simulink model "torque_pi_controller_incremental_algorithm_hardware"  (R2023b)
settings: Solver=FixedStepAuto  StartTime=0.0  StopTime=3.5  RelTol=1e-5  EnableMultiTasking=on
values from neighbouring files (symbols this model uses):
  K = 1.339    [torque_PI_integral_algorithm.m]    (also in torque_PI_tuning.m; torque_model.m = 1.32)
  Kp = pid.Kp    [torque_PI_integral_algorithm.m]    (also in torque_PI_tuning.m = G_T*Ki)
  Ti = pid.Ti    [torque_PI_integral_algorithm.m]    (also in torque_PI_tuning.m = Kp/Ki)
  Ts = 0.005    [torque_PI_integral_algorithm.m]    (also in torque_PI_tuning.m)
undefined symbols (not defined in the file or in its folder): DiscIntNeverNeededParam
settings Model: ExtModeTrigDuration=10  Creator=paoli  LastModifiedBy=kiraa
settings OptimizationCC: EnhancedBackFolding=on  PassReuseOutputArgsAs=Individual arguments  ZeroExternalMemoryAtStartup=off  ZeroInternalMemoryAtStartup=off  MaxStackSize=64  OptimizeBlockOrder=speed  DifferentSizesBufferReuse=on  OptimizationCustomize=off  EfficientTunableParamExpr=on
settings DebuggingCC: ParameterTunabilityLossMsg=error
settings HardwareCC: ProdBitPerPointer=32  ProdBitPerSizeT=32  ProdBitPerPtrDiffT=32  ProdLargestAtomicInteger=Long  ProdLargestAtomicFloat=Double  ProdWordSize=32  ProdLongLongMode=on  ProdHWDeviceType=ARM Compatible->ARM Cortex
settings SFSimCC: MATLABDynamicMemAlloc=off
settings RTWCC: Description=Embedded Coder  SystemTargetFile=ert.tlc  HardwareBoard=STM32 Nucleo F401RE  TemplateMakefile=ert_default_tmf  Toolchain=GNU Tools for ARM Embedded Processors
settings CodeAppCC: ForceParamTrailComments=on  IgnoreCustomStorageClasses=off  OperatorAnnotations=on  SimulinkDataObjDesc=on  SFDataObjDesc=on  InsertBlockDesc=on
settings ERTTargetCC: ExtModeTransport=3  ExtModeStaticAlloc=on  ExtModeStaticAllocSize=2000  ExtModeMexFile=ext_xcp  ExtModeIntrfLevel=Level2 - Open

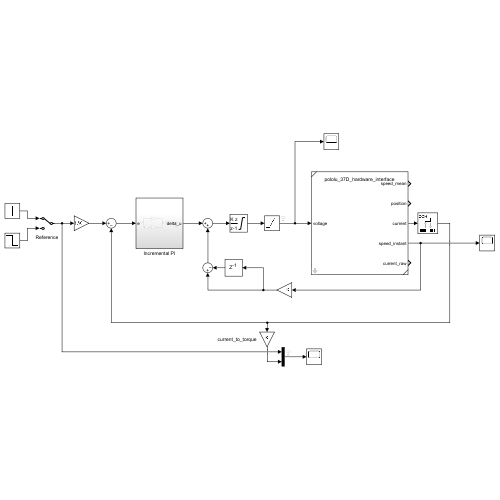
[thumbnail: Simulink's stored preview of the top-level diagram]
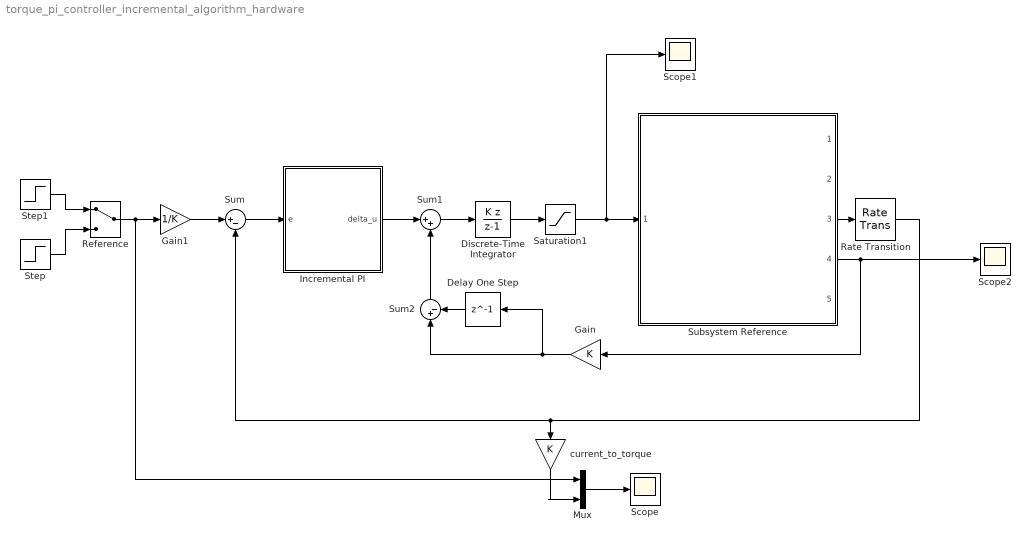
== system torque_pi_controller_incremental_algorithm_hardware ==
  Delay One Step : Delay  DelayLength=1
  Discrete-Time Integrator : DiscreteIntegrator  IntegratorMethod=Accumulation: Backward Euler  SampleTime=-1  LimitOutput=on  UpperSaturationLimit=12  LowerSaturationLimit=-12  ICPrevOutput=DiscIntNeverNeededParam  ICPrevScaledInput=DiscIntNeverNeededParam
  Gain : Gain  Gain=K
  Gain1 : Gain  Gain=1/K
  Incremental PI : Subsystem
  Mux : Mux  Inputs=2
  Rate Transition : RateTransition  OutPortSampleTime=Ts
  Reference : ManualSwitch
  Saturation1 : Saturate  UpperLimit=12  LowerLimit=-12
  Scope : Scope
  Scope1 : Scope
  Scope2 : Scope
  Step : Step  Time=2  Before=1  After=0  SampleTime=Ts
  Step1 : Step  Time=0  After=0.15  SampleTime=Ts
  Subsystem Reference : Subsystem  ReferencedSubsystem=pololu_37D_hardware_interface  Ts=Ts  pwmFreq=2000
  Sum : Sum  Inputs=|+-
  Sum1 : Sum  Inputs=|++
  Sum2 : Sum  Inputs=|+-
  current_to_torque : Gain  Gain=K
  wires:
  Reference/1 -> Gain1/1, Mux/1
  Mux/1 -> Scope/1
  Sum1/1 -> Discrete-Time Integrator/1
  Saturation1/1 -> Scope1/1, Subsystem Reference/1
  Sum/1 -> Incremental PI/1(e)
  Incremental PI/1(delta_u) -> Sum1/1
  Gain/1 -> Sum2/1, Delay One Step/1
  Subsystem Reference/4 -> Scope2/1, Gain/1
  Discrete-Time Integrator/1 -> Saturation1/1
  Sum2/1 -> Sum1/2
  Delay One Step/1 -> Sum2/2
  Subsystem Reference/3 -> Rate Transition/1
  Rate Transition/1 -> Sum/2, current_to_torque/1
  Step/1 -> Reference/2
  Step1/1 -> Reference/1
  Gain1/1 -> Sum/1
  current_to_torque/1 -> Mux/2

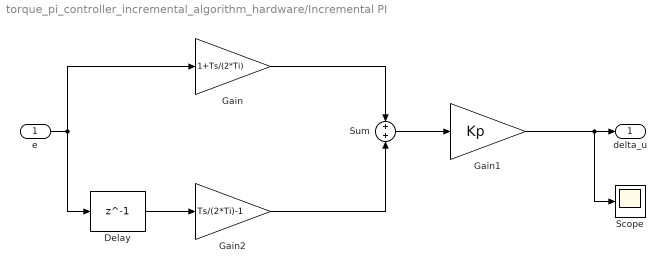
== system torque_pi_controller_incremental_algorithm_hardware/Incremental PI ==
  e : Inport  SampleTime=Ts
  Delay : Delay  DelayLength=1  InitialCondition=0  UseCircularBuffer=on
  Gain : Gain  Gain=1+Ts/(2*Ti)
  Gain1 : Gain  Gain=Kp
  Gain2 : Gain  Gain=Ts/(2*Ti)-1
  Scope : Scope
  Sum : Sum  Inputs=+|+
  delta_u : Outport  SampleTime=Ts
  wires:
  e/1 -> Delay/1, Gain/1
  Delay/1 -> Gain2/1
  Gain/1 -> Sum/1
  Sum/1 -> Gain1/1
  Gain1/1 -> Scope/1, delta_u/1
  Gain2/1 -> Sum/2
